simulink library "gm_FSModem_FPGA_lib"  (R2017b)
settings: Solver=VariableStepAuto  StartTime=0.0  StopTime=10.0  RelTol=1e-3
undefined symbols (not defined in the file): AXI4, F, Lite, sdr
libraries: axiinterfacelib x2
settings Model: Creator=ppradhan  LastModifiedBy=ppradhan

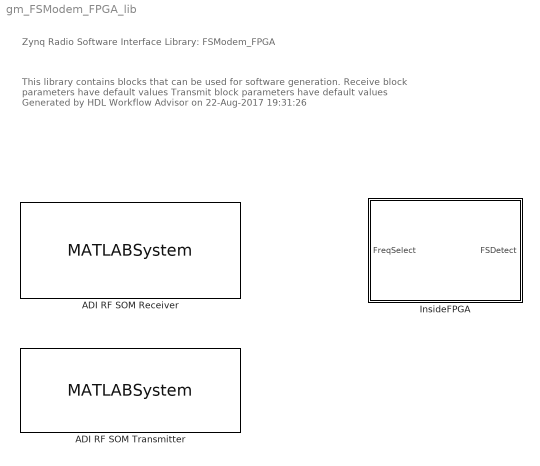
== system gm_FSModem_FPGA_lib ==
  note: Zynq Radio Software Interface Library: FSModem_FPGA
  note: This library contains blocks that can be used for software generation.
      |
      | Receive block parameters have default values
      | Transmit block parameters have default values
      |
      | Generated by HDL Workflow Advisor on 22-Aug-2017 19:31:26
  ADI RF SOM Receiver : MATLABSystem  InitFcn=sdr.internal.registerBlocks(gcb, 'xpicozedsdr');  System=comm.internal.SDRRxADIRFSOMSL  IPAddress=192.168.3.2  CenterFrequencySource=Dialog  CenterFrequency=2400000000  GainSource=AGC Slow Attack  Gain=1  ChannelMapping=1  BasebandSampleRate=3840000  EnableBurstMode=off  NumFramesInBurst=20  OutputDataType=int16  SamplesPerFrame=3660  LostSamplesOutputPort=on  RSSIOutputPort=off  DMATimeoutValue=1  blockMode=Codegen  SimulateUsing=Code generation  EnableQuadratureTracking=on  EnableRFDCTracking=on  EnableBasebandDCTracking=on  BypassUserLogic=off  ShowAdvancedProperties=on  ShowInternalProperties=off  subDeviceList=zynqReceiver  sdrExecutionMode=HW  dataUDPPort=-1  ctrlUDPPort=-1  SourceSelect=RF data  SourceConfiguration1=1023  FIRCoefficientSize=[ 128; 128 ]  FIRCoefficients=[ 55, -54, 42, -126, -123, -317, -399, -581, -646, -711, -634, -507, -263, -10, 255, 424, 492, 401, 201, -84, -352, -540, -566, -423, -126, 234, 562, 738, 701, 429, -5, -490, -866, -1007, -834, -372, 266, 891, 1301, 1334, 936, 178, -733, -1524, -1917, -1731, -944, 274, 1590, 2585, 2881, 2255, 741, -1344, -3435, -4850, -4942, -3285, 197, 5169, 10923, 16509, 20932, 23375, 23375, 20932, 16509, 10923, 5169, 197, -3285, -4942, -4850, -3435, -1344, 741, 2255, 2881, 2585, 1590, 274, -944, -1731, -1917, -1524, -733, 178, 936, 1334, 1301, 891, 266, -372, -834, -1007, -866, -490, -5, 429, 701, 738, 562, 234, -126, -423, -566, -540, -352, -84, 201, 401, 492, 424, 255, -10, -263, -507, -634, -711, -646, -581, -399, -317, -123, -126, 42, -54, 55; 190, -88, 329, -40, 239, -99, -24, -349, -377, -611, -573, -604, -395, -229, 66, 239, 394, 350, 227, -46, -300, -534, -593, -506, -221, 137, 512, 737, 765, 526, 103, -420, -852, -1069, -947, -512, 156, 841, 1341, 1450, 1100, 333, -638, -1531, -2028, -1922, -1152, 115, 1544, 2677, 3099, 2535, 997, -1205, -3479, -5095, -5345, -3750, -199, 4965, 11002, 16895, 21580, 24172, 24172, 21580, 16895, 11002, 4965, -199, -3750, -5345, -5095, -3479, -1205, 997, 2535, 3099, 2677, 1544, 115, -1152, -1922, -2028, -1531, -638, 333, 1100, 1450, 1341, 841, 156, -512, -947, -1069, -852, -420, 103, 526, 765, 737, 512, 137, -221, -506, -593, -534, -300, -46, 227, 350, 394, 239, 66, -229, -395, -604, -573, -611, -377, -349, -24, -99, 239, -40, 329, -88, 190 ]  FIRGain=[ 0; -12 ]  FIRDecimInterpFactor=[ 4; 4 ]  AnalogFilterCutoff=[ 3152524; 3161715 ]  FilterPathRates=[ 983040000, 122880000, 61440000, 30720000, 15360000, 3840000; 983040000, 122880000, 61440000, 30720000, 15360000, 3840000 ]  FilterDesignTypeForTx=DefaultFilterFromOther  FilterDesignTypeForRx=DefaultFilter  BISTLoopbackConfig=No Loopback  BISTPRBSMode=PRBS Disable  BISTToneMode=Tone Disable  BISTToneFrequency=F/32  BISTToneLevel=-6  BISTChannelMask=0  DataIsComplex=on
      mask Type: comm.internal.SDRRxADIRFSOMSL
      mask Display:
      | disp(['ADI RF SOM' char(10) 'ARM-FPGA Interface']);
      | port_label('output',1,'data');
      | port_label('output',2,'data valid');
      | port_label('output',3,'overflow');
  ADI RF SOM Transmitter : MATLABSystem  InitFcn=sdr.internal.registerBlocks(gcb, 'xpicozedsdr');  System=comm.internal.SDRTxADIRFSOMSL  IPAddress=192.168.3.2  CenterFrequencySource=Dialog  CenterFrequency=2400000000  GainSource=Dialog  Gain=-10  ChannelMapping=1  BasebandSampleRate=3840000  EnableBurstMode=off  NumFramesInBurst=20  DMATimeoutValue=1  EnableTxPrimingMode=on  blockMode=Codegen  LostSamplesOutputPort=on  OverflowOutputPort=off  SimulateUsing=Code generation  DataSourceSelect=Host  DDSFrequency=[ 1000000, 1000000; 1000000, 1000000 ]  DDSPhase=[ 0, 0; 0, 0 ]  DDSScale=[ 250000, 250000; 250000, 250000 ]  BypassUserLogic=off  ShowAdvancedProperties=on  ShowInternalProperties=off  subDeviceList=zynqTransmitter  sdrExecutionMode=HW  dataUDPPort=-1  ctrlUDPPort=-1  FIRCoefficientSize=[ 128; 128 ]  FIRCoefficients=[ 55, -54, 42, -126, -123, -317, -399, -581, -646, -711, -634, -507, -263, -10, 255, 424, 492, 401, 201, -84, -352, -540, -566, -423, -126, 234, 562, 738, 701, 429, -5, -490, -866, -1007, -834, -372, 266, 891, 1301, 1334, 936, 178, -733, -1524, -1917, -1731, -944, 274, 1590, 2585, 2881, 2255, 741, -1344, -3435, -4850, -4942, -3285, 197, 5169, 10923, 16509, 20932, 23375, 23375, 20932, 16509, 10923, 5169, 197, -3285, -4942, -4850, -3435, -1344, 741, 2255, 2881, 2585, 1590, 274, -944, -1731, -1917, -1524, -733, 178, 936, 1334, 1301, 891, 266, -372, -834, -1007, -866, -490, -5, 429, 701, 738, 562, 234, -126, -423, -566, -540, -352, -84, 201, 401, 492, 424, 255, -10, -263, -507, -634, -711, -646, -581, -399, -317, -123, -126, 42, -54, 55; 190, -88, 329, -40, 239, -99, -24, -349, -377, -611, -573, -604, -395, -229, 66, 239, 394, 350, 227, -46, -300, -534, -593, -506, -221, 137, 512, 737, 765, 526, 103, -420, -852, -1069, -947, -512, 156, 841, 1341, 1450, 1100, 333, -638, -1531, -2028, -1922, -1152, 115, 1544, 2677, 3099, 2535, 997, -1205, -3479, -5095, -5345, -3750, -199, 4965, 11002, 16895, 21580, 24172, 24172, 21580, 16895, 11002, 4965, -199, -3750, -5345, -5095, -3479, -1205, 997, 2535, 3099, 2677, 1544, 115, -1152, -1922, -2028, -1531, -638, 333, 1100, 1450, 1341, 841, 156, -512, -947, -1069, -852, -420, 103, 526, 765, 737, 512, 137, -221, -506, -593, -534, -300, -46, 227, 350, 394, 239, 66, -229, -395, -604, -573, -611, -377, -349, -24, -99, 239, -40, 329, -88, 190 ]  FIRGain=[ 0; -12 ]  FIRDecimInterpFactor=[ 4; 4 ]  AnalogFilterCutoff=[ 3152524; 3161715 ]  FilterPathRates=[ 983040000, 122880000, 61440000, 30720000, 15360000, 3840000; 983040000, 122880000, 61440000, 30720000, 15360000, 3840000 ]  FilterDesignTypeForTx=DefaultFilter  FilterDesignTypeForRx=DefaultFilterFromOther
      mask Type: comm.internal.SDRTxADIRFSOMSL
      mask Display:
      | disp(['ADI RF SOM' char(10) 'ARM-FPGA Interface']);
      | port_label('input',1,'data');
      | port_label('output',1,'underflow');
      | port_label('output',2,'overflow');
  InsideFPGA : Subsystem  TreatAsAtomicUnit=on  mask(AXI4-Lite/AXI4 Interface){}
      mask help:
      | This is an automatically generated subsystem block.
      | This contains the AXI interface blocks that communicate with the InsideFPG_ip IPCore generated from FSModem_FPGA/InsideFPGA subsystem.
      mask Display: disp(sprintf('Xilinx Zynq \nAXI Interface'));

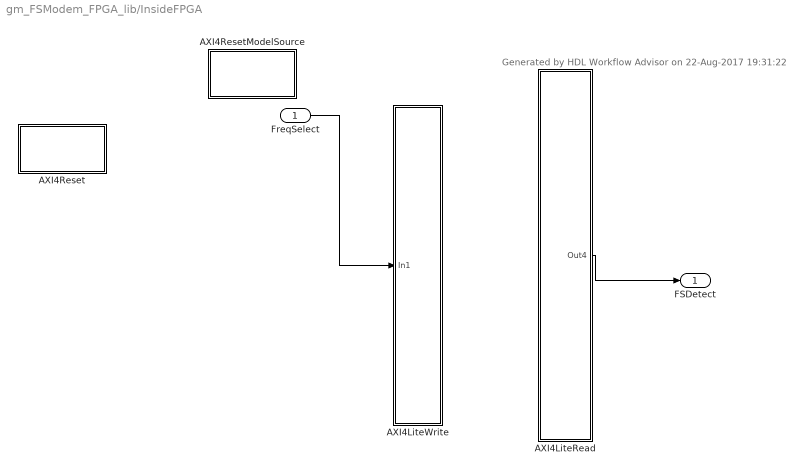
== system gm_FSModem_FPGA_lib/InsideFPGA ==
  note: Generated by HDL Workflow Advisor on 22-Aug-2017 19:31:22
  FreqSelect : Inport
  AXI4LiteRead : Subsystem  Priority=10
  AXI4LiteWrite : Subsystem  Priority=1
  AXI4Reset : Subsystem  mask(System Start){ShowInLibBrowser=0}
      mask prompts: ShowInLibBrowser "Simulink:masks:CustCodeMaskParam1_MP"
      settings: CopyFcn=cccopyfcn(gcb)  OpenFcn=ccopenfcn('System Start Function')
      mask Help: eval('feval(''rtwprivate'',''rtwhelpview'',''rtw_sys_start_block'')');
      mask Display: disp('System\nStart');
  AXI4ResetModelSource : Subsystem  mask(Model Source){ShowInLibBrowser=0}
      mask prompts: ShowInLibBrowser "Simulink:masks:CustCodeMaskParam1_MP"
      settings: CopyFcn=cccopyfcn(gcb)  OpenFcn=ccopenfcn('Model Source')
      mask Help: eval('feval(''rtwprivate'',''rtwhelpview'',''rtw_model_source_block'')');
      mask Display: disp('Model\nSource');
  FSDetect : Outport
  wires:
  AXI4LiteRead/1(Out4) -> FSDetect/1
  FreqSelect/1 -> AXI4LiteWrite/1(In1)

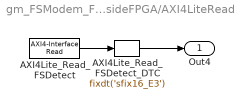
== system gm_FSModem_FPGA_lib/InsideFPGA/AXI4LiteRead ==
  AXI4Lite_Read_FSDetect : axiinterfacelib/AXI4-Interface Read  Priority=2  AXIInterfaceType=AXI4-Lite  DeviceName=/dev/mwipcore1  RegisterOffset=hex2dec('104')  DataLength=1  DataType=uint32  SampleTime=-1  blockPlatform=ZYNQ  SimulateUsing=Interpreted Execution
      settings: SourceProductName=Embedded Coder Support Package for Xilinx Zynq Platform  SourceProductBaseCode=ECZYNQ7000
  AXI4Lite_Read_FSDetect_DTC : DataTypeConversion  OutDataTypeStr=fixdt('sfix16_E3')  ConvertRealWorld=Stored Integer (SI)
  Out4 : Outport
  wires:
  AXI4Lite_Read_FSDetect/1 -> AXI4Lite_Read_FSDetect_DTC/1
  AXI4Lite_Read_FSDetect_DTC/1 -> Out4/1

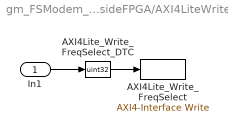
== system gm_FSModem_FPGA_lib/InsideFPGA/AXI4LiteWrite ==
  In1 : Inport
  AXI4Lite_Write_FreqSelect : axiinterfacelib/AXI4-Interface Write  Priority=1  AXIInterfaceType=AXI4-Lite  DeviceName=/dev/mwipcore1  RegisterOffset=hex2dec('100')  blockPlatform=ZYNQ  SimulateUsing=Interpreted execution
      settings: SourceProductName=Embedded Coder Support Package for Xilinx Zynq Platform  SourceProductBaseCode=ECZYNQ7000
  AXI4Lite_Write_FreqSelect_DTC : DataTypeConversion  OutDataTypeStr=uint32  ConvertRealWorld=Stored Integer (SI)
  wires:
  AXI4Lite_Write_FreqSelect_DTC/1 -> AXI4Lite_Write_FreqSelect/1
  In1/1 -> AXI4Lite_Write_FreqSelect_DTC/1

== system gm_FSModem_FPGA_lib/InsideFPGA/AXI4Reset ==

== system gm_FSModem_FPGA_lib/InsideFPGA/AXI4ResetModelSource ==
